simulink model "NHS_speaker_adaptive_notch_filter_showcase_1024nfft_buffer"  (R2022b)
settings: Solver=FixedStepDiscrete  StartTime=0.0  StopTime=inf  RelTol=1e-3
libraries: simulink x2, audiosources x1, dspsnks4 x1, dspxfrm3 x1, dspvision x1, dspfdesign x1
settings Model: Creator=zhouyiliang  LastModifiedBy=zhouyiliang
settings SolverCC: AlgebraicLoopSolver=TrustRegion  AutoInsertRateTranBlk=on
settings DataIOCC: LimitDataPoints=on  SaveOutput=off  SignalLogging=off  SaveTime=off
settings OptimizationCC: LifeSpan=inf
settings DebuggingCC: AlgebraicLoopMsg=error  SingleTaskRateTransMsg=error  UnconnectedInputMsg=warning  UnconnectedOutputMsg=warning  UnconnectedLineMsg=warning  AllowSymbolicDim=off  SFUnexpectedBacktrackingDiag=warning  SFNoUnconditionalDefaultTransitionDiag=warning  SFExecutionAtInitializationDiag=none  SFMachineParentedDataDiag=warning  ArithmeticOperatorsInVariantConditions=warning
settings ModelReferenceCC: EnableRefExpFcnMdlSchedulingChecks=on
settings SFSimCC: SimUseLocalCustomCode=off  CustomCodeUndefinedFunction=UseInterfaceOnly
settings RTWCC: RTWUseLocalCustomCode=off  DLArmComputeVersion=19.05
settings CodeAppCC: StateflowObjectComments=on
settings GRTTargetCC: TargetLangStandard=C89/C90 (ANSI)
settings ConfigComp: CovMetricSettings=dw  CovSaveCumulativeToWorkspaceVar=on  CovSaveSingleToWorkspaceVar=on  CovExternalEMLEnable=off  CovSFcnEnable=off

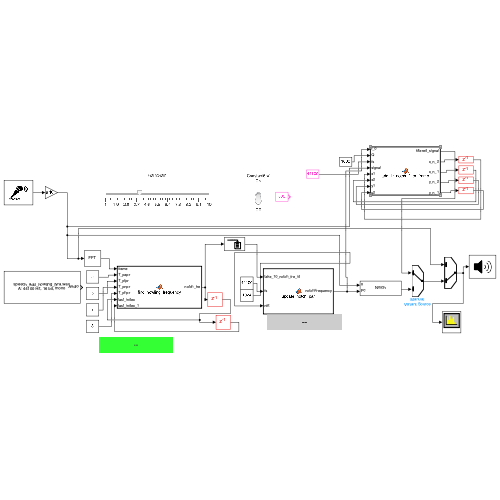
[thumbnail: Simulink's stored preview of the top-level diagram]
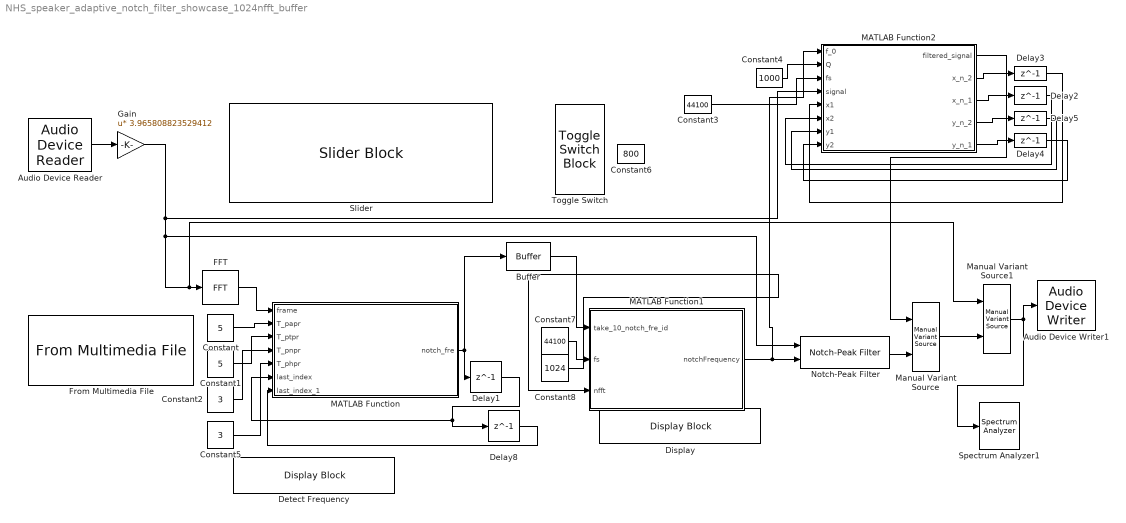
== system NHS_speaker_adaptive_notch_filter_showcase_1024nfft_buffer ==
  Audio Device Reader : audiosources/Audio Device Reader  Driver=CoreAudio  Device=Default  SampleRate=44100  NumChannels=1  SamplesPerFrame=882  BitDepth=16-bit integer  NumBuffers=10  DefaultInputChannelMapping=on  InputChannelMapping=1:2  OutputNumOverrunSamples=off  OutputDataType=double  DriverIdx=5  DeviceWarnFlag=M-Track 2X2M
  Audio Device Writer1 : dspsnks4/Audio Device Writer  Driver=CoreAudio  Device=Default  InheritSampleRate=on  SampleRate=44100  BitDepth=16-bit integer  BufferSize=4096  NumBuffers=10  DefaultOutputChannelMapping=on  OutputChannelMapping=1:2  OutputNumUnderrunSamples=off  DriverIdx=5  DeviceWarnFlag=M-Track 2X2M
  Buffer : Buffer  N=1  OutputFrames=off
  Constant : Constant  Value=5
  Constant1 : Constant  Value=5
  Constant2 : Constant  Value=3
  Constant3 : Constant  Value=44100
  Constant4 : Constant  Value=1000
  Constant5 : Constant  Value=3
  Constant6 : Constant  Value=800
  Constant7 : Constant  Value=44100
  Constant8 : Constant  Value=1024
  Delay{1..5,8} (6 alike) : Delay  DelayLength=1  InitialCondition=0
  "Detect Frequency " : DisplayBlock  LabelPosition=Hide  Transparency=1
  Display : DisplayBlock  LabelPosition=Hide  Transparency=1
  FFT : dspxfrm3/FFT  FFTImplementation=Auto  CompMethod=Table lookup  TableOpt=NEW  TableOptActive=Speed  BitRevOrder=off  Normalize=off  InheritFFTLength=off  FFTLength=1024  WrapInput=on  roundingMode=Floor  overflowMode=off  firstCoeffDataTypeStr=Inherit: Same word length as input  firstCoeffLastDataTypeStr=Inherit: Same word length as input  outputMin=[]  outputMax=[]
  From Multimedia File : dspvision/From Multimedia File  inputFilename=/Users/zhouyiliang/Desktop/work/sound_output/speech_add_howling_fyra.wav  readRange=[1 Inf]  loop=on  numPlays=inf  outputStreams=Audio only  videoDataType=single  audioDataType=double  inheritSampleTime=on  userDefinedSampleTime=1/30  noAudioOutput=off  isIntensityVideo=off  fourcc=RGB  colorVideoFormat=Separate color signals  outputEOF=off  dataOrg=Column-major  audioFrameSize=882  computeAudioFrameSize=off  outSamplingMode=Sample based
  Gain : Gain  Gain=3.965808823529412  Multiplication=Matrix(u*K)
  MATLAB Function : MATLAB Function  TreatAsAtomicUnit=on
  MATLAB Function1 : MATLAB Function  TreatAsAtomicUnit=on
  MATLAB Function2 : MATLAB Function  TreatAsAtomicUnit=on
  Manual Variant Source : simulink/Signal Routing/Manual Variant Source  NumChoices=2  LabelModeActiveChoice=V_1
  Manual Variant Source1 : simulink/Signal Routing/Manual Variant Source  NumChoices=2  LabelModeActiveChoice=V_2
  Notch-Peak Filter : dspfdesign/Notch-Peak Filter  Specification=Quality factor and center frequency  BandwidthPort=off  Bandwidth=2205  QualityFactorPort=off  QualityFactor=1  CenterFrequencyPort=on  CenterFrequency=11025  BandwidthCoefficientPort=off  BandwidthCoefficient=0.72654  CenterFrequencyCoefficientPort=off  CenterFrequencyCoefficient=0  Output=Notch  InheritSampleRate=off  SampleRate=44100  SimulateUsing=Code generation
  Slider : SliderBlock  ScaleMin=1  ScaleMax=10
  Spectrum Analyzer1 : SpectrumAnalyzer
  Toggle Switch : ToggleSwitchBlock
      settings: Values={{'Off', 'On'}, [800 2000]}
  wires:
  FFT/1 -> MATLAB Function/1(frame)
  Constant/1 -> MATLAB Function/2(T_papr)
  Constant1/1 -> MATLAB Function/3(T_ptpr)
  Constant2/1 -> MATLAB Function/4(T_pnpr)
  Constant5/1 -> MATLAB Function/5(T_phpr)
  Manual Variant Source/1 -> Manual Variant Source1/2
  Delay1/1 -> Delay8/1, MATLAB Function/6(last_index)
  Notch-Peak Filter/1 -> Manual Variant Source/2
  MATLAB Function2/1(filtered_signal) -> Manual Variant Source/1
  Constant7/1 -> MATLAB Function1/2(fs)
  Constant8/1 -> MATLAB Function1/3(nfft)
  MATLAB Function1/1(notchFrequency) -> MATLAB Function2/1(f_0), Notch-Peak Filter/2
  MATLAB Function2/3(x_n_1) -> Delay2/1
  MATLAB Function2/2(x_n_2) -> Delay3/1
  MATLAB Function2/5(y_n_1) -> Delay4/1
  MATLAB Function2/4(y_n_2) -> Delay5/1
  Delay2/1 -> MATLAB Function2/6(x2)
  Delay3/1 -> MATLAB Function2/5(x1)
  Delay5/1 -> MATLAB Function2/7(y1)
  Delay4/1 -> MATLAB Function2/8(y2)
  MATLAB Function/1(notch_fre) -> Delay1/1, Buffer/1
  Delay8/1 -> MATLAB Function/7(last_index_1)
  Constant3/1 -> MATLAB Function2/3(fs)
  Constant4/1 -> MATLAB Function2/2(Q)
  Manual Variant Source1/1 -> Spectrum Analyzer1/1, Audio Device Writer1/1
  Gain/1 -> Manual Variant Source1/1, FFT/1, Notch-Peak Filter/1, MATLAB Function2/4(signal)
  Buffer/1 -> MATLAB Function1/1(take_10_notch_fre_id)
  Audio Device Reader/1 -> Gain/1

== matlab function NHS_speaker_adaptive_notch_filter_showcase_1024nfft_buffer/MATLAB Function1 ==
  data: take_10_notch_fre_id input; notchFrequency output; fs input; nfft input
function notchFrequency = update_notch_par(take_10_notch_fre_id, fs, nfft)
    current_notch_fre_id = 2;
    if any(take_10_notch_fre_id == 2)
        notchFrequency = 0;
    else
        % 计算A中每个元素出现的次数
        [counts, bins] = histcounts(take_10_notch_fre_id);

        % 找到出现次数最大的元素的索引
        [max_count, max_idx] = max(counts);

        % 判断最大出现次数是否大于等于3，如果是，则将b赋值为对应的元素
        if max_count >= 1
            current_notch_fre_id = bins(max_idx);
        else
            current_notch_fre_id = 1;
        end
    
        freqs = linspace(0, fs, nfft);
    %     if current_notch_fre_id == 0 
    %         current_notch_fre_id = 2 ;
    %     end
        if current_notch_fre_id > 0 && current_notch_fre_id <= length(freqs)
        notchFrequency = floor(floor(max(freqs(current_notch_fre_id+1) + 20, 0)));
        else
            notchFrequency = 0;
        end
    end
end

== matlab function NHS_speaker_adaptive_notch_filter_showcase_1024nfft_buffer/MATLAB Function ==
  data: frame input; T_papr input; T_ptpr input; T_pnpr input; T_phpr input; last_index input; notch_fre output; last_index_1 input
function notch_fre = find_howling_frequency(frame, T_papr, T_ptpr, T_pnpr,T_phpr,last_index, last_index_1)
    
%%%%%Args:
        %frame: Spectrum of one frame.
        %T_...: Power threshold value in dB for different methods.
    %Returns:
        %Notch Frequency for current frame
    power = abs(frame).^2;
    papr = zeros(length(power),1);
    avarage = mean(power);
    ret_papr = [];
    ret_ptpr = [];
    ret_pnpr = [];
    ret_phpr = [];
    for i = 4:1:length(frame)-3 % take 4:end-3
        papr(i) = 10*log10(power(i)/avarage) ;
%%%%% Peak-to-Avarage Power Ratio (PAPR)
        if papr(i) > T_papr
            ret_papr = [ret_papr, i];
        end
%%%%% Peak-to-Threshold Power Ratio (PTPR)
        if (10*log10(power(i)) > T_ptpr)
            ret_ptpr = [ret_ptpr, i];
        end
%%%%% Peak-to-Neighboring Power Ratio (PNPR)
        if (10*log10(power(i)/power(i-2)) > T_pnpr) ...
            && (10*log10(power(i)/power(i-3)) > T_pnpr)...
            && (10*log10(power(i)/power(i+2)) > T_pnpr )...
            && (10*log10(power(i)/power(i+3)) > T_pnpr)
            ret_pnpr = [ret_pnpr, i];
        end
    end
    % %%%%% Peak-to-Harmonic Power Ratio (PHPR)
    for i = 1:1:floor(length(frame)/3)
        if (10*log10(power(i)/power(2*i)) > T_phpr) && (10*log10(power(i)/power(3*i)) > T_phpr)
            ret_phpr = [ret_phpr, i];
        end
    end
    
    % interselect 
    
    fre_index = intersect(intersect(intersect(ret_papr,ret_ptpr,'stable'),ret_pnpr,'stable'),ret_phpr,'stable');
    if ~isempty(fre_index) 
        fre_index_1 = min(fre_index);
    else
%         fre_index_1 = fre_index_1+1;
        fre_index_1 = 1;
    end

    if fre_index_1 ~= last_index && fre_index_1 ~= last_index_1 
        notch_fre = fre_index_1;
    else
        notch_fre = last_index;
    end
%     choose stable filter index
    flag = [0
1
0
1
0
0
1
0
1
0
0
1
0
1
0
0
1
0
1
0
0
1
0
1
0
0
1
0
1
0
0
1
0
1
0
0
1
0
1
0
0
1
0
1
0
0
1
0
1
0
0
1
0
1
1
0
1
0
1
1
0
1
0
1
1
0
1
0
1
1
0
1
0
1
1
0
1
0
1
1
0
1
0
1
1
0
1
0
1
1
0
1
0
1
1
0
1
0
1
1
0
1
0
1
1
0
1
0
0
1
0
1
0
0
1
0
1
0
0
1
0
1
0
0
1
0
1
0
0
1
0
1
0
0
1
0
1
0
0
1
0
1
0
0
1
0
1
0
0
1
0
1
0
0
1
0
1
0
0
1
0
1
1
0
1
0
1
1
0
1
0
1
1
0
1
0
1
1
0
1
0
1
1
0
1
0
1
1
0
1
0
1
1
0
1
0
1
1
0
1
0
1
1
0
1
0
1
1
0
1
0
1
1
0
1
0
0
1
0
1
0
0
1
0
1
0
0
1
0
1
0
0
1
0
1
0
0
1
0
1
0
0
1
0
1
0
0
1
0
1
0
0
1
0
1
0
0
1
0
1
0
0
1
0
1
1
0
1
0
1
1
0
1
0
1
1
0
1
0
1
1
0
1
0
1
1
0
1
0
1
1
0
1
0
1
1
0
1
0
1
1
0
1
0
1
1
0
1
0
1
1
0
1
0
1
1
0
1
0
0
1
0
1
0
0
1
0
1
0
0
1
0
1
0
0
1
0
1
0
0
1
0
1
0
0
1
0
1
0
0
1
0
1
0
0
1
0
1
0
0
1
0
1
0
0
1
0
1
0
0
1
0
1
1
0
1
0
1
1
0
1
0
1
1
0
1
0
1
1
0
1
0
1
1
0
1
0
1
1
0
1
0
1
1
0
1
0
1
1
0
1
0
1
1
0
1
0
1
1
0
1
0
1
1
0
1
0
0
1
0
1
0
0
1
0
1
0
0
1
0
1
0
0
1
0
1
0
0
1
0
1
0
0
1
0
1
0
0
1
0
1
0
0
1
0
1
0
0
1
0
1
0
0
1
0
1
0
0
1
0
1
1
0
1
0
1
1
0
1
0
1
1
0
1
0
1
1
0
1
0
1
1
0
1
0
1
1
0
1
0
1
1
0
1
0
1
1
0
1
0
1
1
0
1
0
1
1
0
1
0
0
1
0
1
0
0
1
0
1
0
0
1
0
1
0
0
1
0
1
0
0
1
0
1
0
0
1
0
1
0
0
1
0
1
0
0
1
0
1
0
0
1
0
1
0
0
1
0
1
0
0
1
0
1
1
0
1
0
1
1
0
1
0
1
1
0
1
0
1
1
0
1
0
1
1
0
1
0
1
1
0
1
0
1
1
0
1
0
1
1
0
1
0
1
1
0
1
0
1
1
0
1
0
1
1
0
1
0
0
1
0
1
0
0
1
0
1
0
0
1
0
1
0
0
1
0
1
0
0
1
0
1
0
0
1
0
1
0
0
1
0
1
0
0
1
0
1
0
0
1
0
1
0
0
1
0
1
0
0
1
0
1
1
0
1
0
1
1
0
1
0
1
1
0
1
0
1
1
0
1
0
1
1
0
1
0
1
1
0
1
0
1
1
0
1
0
1
1
0
1
0
1
1
0
1
0
1
1
0
1
0
1
1
0
1
0
0
1
0
1
0
0
1
0
1
0
0
1
0
1
0
0
1
0
1
0
0
1
0
1
0
0
1
0
1
0
0
1
0
1
0
0
1
0
1
0
0
1
0
1
0
0
1
0
1
1
0
1
0
1
1
0
1
0
1
1
0
1
0
1
1
0
1
0
1
1
0
1
0
1
1
0
1
0
1
1
0
1
0
1
1
0
1
0
1
1
0
1
0
1
1
0
1
0
1
1
0
1
0
0
1
0
1
0
0
1
0
1
0
0
1
0
1
0
0
1
0
1
0
0
1
0
1
0
0
1
0
1
0
0
1
0
1
0
0
1
0
1
0
0
1
0
1
0
0
1
0
1
0
0
1
0
1
1
0
1
0
1
1
0
1
0
1
1
0
1
0
1
1
0
1
0
1
1
0
1
0
1
1
0
1
0
1
1
0
1
0
1
1
0
1
0
1
1
0
1
0
1
1
0
1
0
1
1
0
1
0
0
1
0
1
0
0
1
0
1
0
0
1
0
1
0
0
1
0
1
0
0
1
0
1
0
0
1
0
1
0
0
1
0
1
0
0
1
0
1
0
0
1
0
1
0
0
1
0
1
0
0
1
0
1
1
0
1
0
1
1
0
1
0
1
1
0
1
0
1
1
0
1
0
1
1
0
1
0
1
1
0
1
0
1
1
0
1
0
1
1
0
1
0
1
1
0
1
0
1
1
0
1
0
0
1
0
1
0
0
1
0
1
0
0
1
0
1
0
0
1
0
1
0
0
1
0
1
0
0
1
0
1
0
0
1
0
1
0
0
1
0
1
0
0
1
0
1
0
0
1
0
1
0
0
1
0
1
1
0
1
0
1
1
0
1
0
1
1
0
1
0
1
1
0
1
0
1
1
0
1
0
1
1
0
1
0
1
1
0
1
0
1
1
0
1
0
1
1
0
1
0
1
1
0
1
0
1
1
0
1
0
0
1
0
1
0
0
1
0
1
0
0
1
0
1
0
0
1
0
1
0
0
1
0
1
0
0
1
0
1
0
0
1
0
1
0
0
1
0
1
0
0
1
0
1
0
0
1
0
1
0
0
1
0
1
1
0
1
0
1
1
0
1
0
1
1
0
1
0
1
1
0
1
0
1
1
0
1
0
1
1
0
1
0
1
1
0
1
0
1
1
0
1
0
1
1
0
1
0
1
1
0
1
0
1
1
0
1
0
0
1
0
1
0
0
1
0
1
0
0
1
0
1
0
0
1
0
1
0
0
1
0
1
0
0
1
0
1
0
0
1
0
1
0
0
1
0
1
0
0
1
0
1
0
0
1
0
1
1
0
1
0
1
1
0
1
0
1
1
0
1
0
1
1
0
1
0
1
1
0
1
0
1
1
0
1
0
1
1
0
1
0
1
1
0
1
0
1
1
0
1
0
1
1
0
1
0
1
1
0
1
0
0
1
0
1
0
0
1
0
1
0
0
1
0
1
0
0
1
0
1
0
0
1
0
1
0
0
1
0
1
0
0
1
0
1
0
0
1
0
1
0
0
1
0
1
0
0
1
0
1
0
0
1
0
1
1
0
1
0
1
1
0
1
0
1
1
0
1
0
1
1
0
1
0
1
1
0
1
0
1
1
0
1
0
1
1
0
1
0
1
1
0
1
0
1
1
0
1
0
1
1
0
1
0
1
1
0
1
0
0
1
0
1
0
0
1
0
1
0
0
1
0
1
0
0
1
0
1
0
0
1
0
1
0
0
1
0
1
0
0
1
0
1
0
0
1
0
1
0
0
1
0
1
0
0
1
0
1
0
0
1
0
1
1
0
1
0
1
1
0
1
0
1
1
0
1
0
1
1
0
1
0
1
1
0
1
0
1
1
0
1
0
1
1
0
1
0
1
1
0
1
0
1
1
0
1
0
1
1
0
1
0
0
1
0
1
0
0
1
0
1
0
0
1
0
1
0
0
1
0
1
0
0
1
0
1
0
0
1
0
1
0
0
1
0
1
0
0
1
0
1
0
0
1
0
1
0
0
1
0
1
0
0
1
0
1
1
0
1
0
1
1
0
1
0
1
1
0
1
0
1
1
0
1
0
1
1
0
1
0
1
1
0
1
0
1
1
0
1
0
1
1
0
1
0
1
1
0
1
0
1
1
0
1
0
1
1
0
1
0
0
1
0
1
0
0
1
0
1
0
0
1
0
1
0
0
1
0
1
0
0
1
0
1
0
0
1
0
1
0
0
1
0
1
0
0
1
0
1
0
0
1
0
1
0
0
1
0
1
0
0
1
0
1
1
0
1
0
1
1
0
1
0
1
1
0];

if flag(notch_fre) == 0
    while notch_fre < length(flag)
        notch_fre = notch_fre + 1;
        if flag(notch_fre) == 1
            break
        end
    end
end
end

== matlab function NHS_speaker_adaptive_notch_filter_showcase_1024nfft_buffer/MATLAB Function2 ==
  data: f_0 input; Q input; fs input; filtered_signal output; x_n_2 output; signal input; x1 input; x2 input; x_n_1 output; y_n_2 output; y1 input; y2 input; y_n_1 output
function [filtered_signal,x_n_2, x_n_1, y_n_2, y_n_1] = add_iir_notch_filter_frame(f_0, Q, fs,signal, x1 ,x2, y1, y2)
    % ARG: f_0 center Frequency, Q: quality factor, fs: sampling frequency,
    % original signal
    % RETURN: filtered signal 
    if f_0 == 0
        x_n_1 = signal(end);%x(n-1)
        x_n_2 = signal(end-1); %x(n-2)
        y = [y1; y2 ;signal];
        filtered_signal=y(3:884);
        y_n_2 = y(end-1); %the one before last, y(n-2)
        y_n_1 = y(end); %last sample , y(n-1)
    else
        x_n_1 = signal(end);%x(n-1)
        x_n_2 = signal(end-1); %x(n-2)
        dw = 1; %3 dB bandwidth
        w_0 = 2*pi*f_0/fs;
        b = 1/(1+tan(dw/2)); % formula reference: help dsp.NotchPeakFilter
%         notch_b = b * [1, -2*cos(w_0) ,1]; %numerator
%         notch_a = [1, -2*b*cos(w_0), 2*b-1]; %denominator 
        N=length(signal);
        x = [x1 ;x2;signal];
        y = zeros(length(signal),1);
        y = [y1; y2 ;y];
           
        mu = 0.001;
        for k=1:N
            %%%% sng-sng LMS %%%%% to get optimized b
            %ADAPTIVE HOWLING CANCELLER USING ADAPTIVE IIR NOTCH FILTER: SIMULATION AND IMPLIMENTATION 
            %W. Leotwassana, R. Punchalard, and K Silaphan  
            notch_b = b * [1, -2*cos(w_0) ,1]; %numerator
            notch_a = [1, -2*b*cos(w_0), 2*b-1]; %denominator 
            W = [notch_b,-notch_a(2:3)]'; % notch filter coefficients
            y(k+2) = [x(k+2) x(k+1) x(k) y(k+1) y(k)] * W;%convolution with filter coefficients
            w = [1 (-0.95)]';
            g = [y(k+2) x(k+2)] * w; %g(n) is the gradient signal, g>0 the signal is increasing
            dw = dw + mu * sign(sign(abs(y(k+1))-abs(y(k)))*g); % dw decrease , filter is with less amplitue
            dw = min(dw,0.4*pi);
            dw = max(dw, 0.001);
            b = 1/(1+tan(dw/2));
            
        end
        filtered_signal=y(3:884);
        y_n_2 = y(end-1); %the one before last, y(n-2)
        y_n_1 = y(end); %last sample , y(n-1)
    
    end
end
